simulink model "peproj2"  (R2025a)
settings: Solver=FixedStepAuto  StartTime=0.0  StopTime=0.07  FixedStep=1e-6  RelTol=1e-3
settings Model: Creator=Hp  LastModifiedBy=Hp

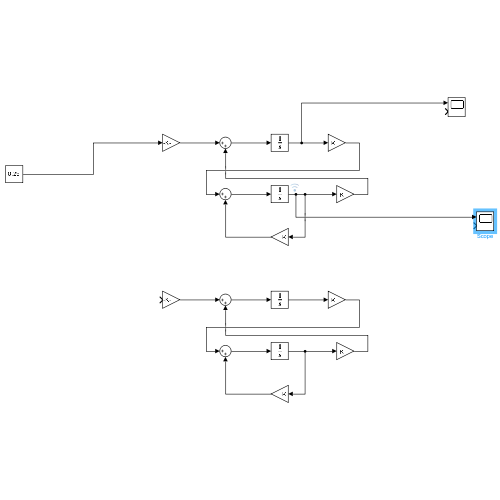
[thumbnail: Simulink's stored preview of the top-level diagram]
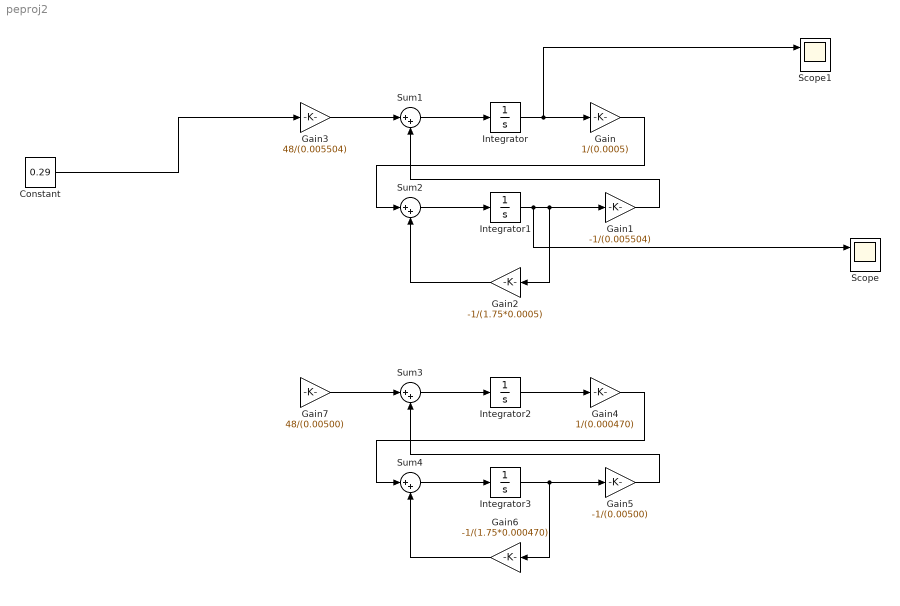
== system peproj2 ==
  Constant : Constant  Value=0.29
  Gain : Gain  Gain=1/(0.0005)
  Gain1 : Gain  Gain=-1/(0.005504)
  Gain2 : Gain  Gain=-1/(1.75*0.0005)
  Gain3 : Gain  Gain=48/(0.005504)
  Gain4 : Gain  Gain=1/(0.000470)
  Gain5 : Gain  Gain=-1/(0.00500)
  Gain6 : Gain  Gain=-1/(1.75*0.000470)
  Gain7 : Gain  Gain=48/(0.00500)
  Integrator{,1..3} (4 alike) : Integrator
  Scope : Scope  NumInputPorts=2
      settings: ActiveDisplayYMinimum=2.1953980176209473  ActiveDisplayYMaximum=16.410155596113945
  Scope1 : Scope  NumInputPorts=2
      settings: ActiveDisplayYMinimum=-1.2761097370914065  ActiveDisplayYMaximum=12.521084680842991
  Sum{1..4} (4 alike) : Sum  Inputs=|++
  wires:
  Gain3/1 -> Sum1/1
  Sum1/1 -> Integrator/1
  Integrator/1 -> Scope1/1, Gain/1
  Gain/1 -> Sum2/1
  Integrator1/1 -> Scope/1, Gain2/1, Gain1/1
  Gain1/1 -> Sum1/2
  Sum2/1 -> Integrator1/1
  Gain2/1 -> Sum2/2
  Gain7/1 -> Sum3/1
  Integrator2/1 -> Gain4/1
  Gain5/1 -> Sum3/2
  Gain4/1 -> Sum4/1
  Gain6/1 -> Sum4/2
  Integrator3/1 -> Gain5/1, Gain6/1
  Sum4/1 -> Integrator3/1
  Sum3/1 -> Integrator2/1
  Constant/1 -> Gain3/1
